simulink library "Brakes_Axle2_HydraulicValves_Channel4"  (R2026a)
settings: Solver=VariableStepAuto
undefined symbols (not defined in the file): Brakes
libraries: fl_lib x32, nesl_utility x18, SimscapeFluids_lib x8, sdl_lib x4, Brakes_Elements x4
(part 1 of 2)
Description:
  | Component of Simscape Vehicle Templates Library
  | 
  | Copyright 2018-2026 The MathWorks, Inc.
settings Model: Creator=smiller  LastModifiedBy=smiller

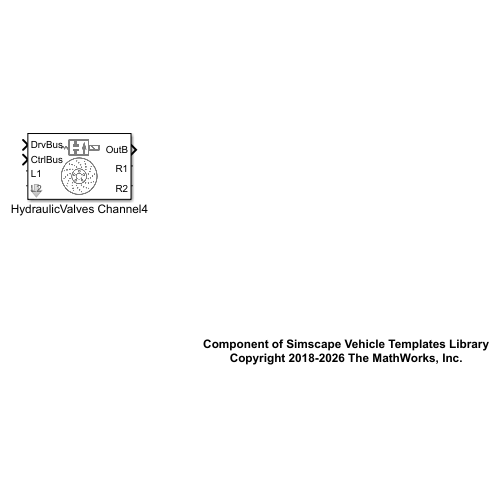
[thumbnail: Simulink's stored preview of the top-level diagram]
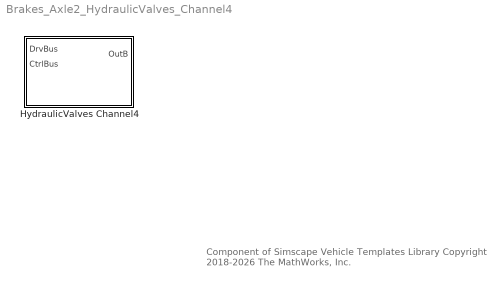
== system Brakes_Axle2_HydraulicValves_Channel4 ==
  note: Component of Simscape Vehicle Templates Library
      | Copyright 2018-2026 The MathWorks, Inc.
  HydraulicValves Channel4 : Subsystem  Tag=PublishSubsystem  VariantControl=ABS_4_Channel  mask(Four Channel ABS){d_caliper_bore_a1=Brakes.Axle1.Caliper.lCylinderDiameter.Value, d_caliper_bore_a2=Brakes.Axle2.Caliper.lCylinderDiameter.Value, brk_pad_rad_a1=Brakes.Axle1.DiscAndPad.lMeanRadius.Value, brk_pad_rad_a2=Brakes.Axle2.DiscAndPad.lMeanRadius.Value, brk_cyl_bore_a1=Brakes.Axle1.Caliper.lCylinderDiameter.Value, brk_cyl_bore_a2=Brakes.Axle2.Caliper.lCylinderDiameter.Value, brk_n_pads_a1=Brakes.Axle1.DiscAndPad.NPads.Value, brk_n_pads_a2=Brakes.Axle2.DiscAndPad.NPads.Value, brk_mu_static_a1=Brakes.Axle1.DiscAndPad.rMuStatic.Value, brk_mu_static_a2=Brakes.Axle2.DiscAndPad.rMuStatic.Value, brk_mu_kin_a1=Brakes.Axle1.DiscAndPad.rMuKinetic.Value, brk_mu_kin_a2=Brakes.Axle2.DiscAndPad.rMuKinetic.Value, brk_trans_vel_a1=Brakes.Axle1.DiscAndPad.nTransition.Value, brk_trans_vel_a2=Brakes.Axle2.DiscAndPad.nTransition.Value, brk_visc_coef_a1=Brakes.Axle1.DiscAndPad.dViscous.Value, brk_visc_coef_a2=Brakes.Axle2.DiscAndPad.dViscous.Value, spr_rate=Brakes.Axle1.ValveApply.kSpring.Value, D=Brakes.Axle1.ValveApply.bDamper.Value, area_max_apply=Brakes.Axle1.ValveApply.AMax.Value, open_max_apply=Brakes.Axle1.ValveApply.xMax.Value, area_max_rel=Brakes.Axle1.ValveRelease.AMax.Value, open_max_rel=Brakes.Axle1.ValveRelease.xMax.Value, p_max_a1=Brakes.Axle1.Caliper.pMax.Value, p_max_a2=Brakes.Axle2.Caliper.pMax.Value, brkTs=Brakes.Axle1.ValveApply.fValveTime.Value}
      mask prompts: spr_rate "Spring Rate (N/m)"; D "Damping coefficient"; area_max_apply "Max Area Apply Valve (m^2)"; open_max_apply "Max Opening Apply Valve (m)"; area_max_rel "Max Area Release Valve (m^2)"; open_max_rel "Max Opening Release Valve (m)"; p_max_a1 "Max Master Cylinder Pressure Axle 1 (bar)"; p_max_a2 "Max Master Cylinder Pressure Axle 2 (bar)"; brkTs "Filter time constant"
      mask help: Models braking system for four wheels. Valve signals control hydraulic pressure at each wheel individually.
      mask init:
      | pist_area_pist_a1 = pi*d_caliper_bore_a1^2/4;
      | pist_area_pist_a2 = pi*d_caliper_bore_a2^2/4;
      mask TypeOptions brk_pad_rad_a1:
      | Disc
      | Brake
      | L1/r_mean | Disc
      | Brake
      | R1/r_mean
      mask TypeOptions brk_pad_rad_a2:
      | Disc
      | Brake
      | L2/r_mean | Disc
      | Brake
      | R2/r_mean
      mask TypeOptions brk_cyl_bore_a1:
      | Disc
      | Brake
      | L1/bore | Disc
      | Brake
      | R1/bore
      mask TypeOptions brk_cyl_bore_a2:
      | Disc
      | Brake
      | L2/bore | Disc
      | Brake
      | R2/bore
      mask TypeOptions brk_n_pads_a1:
      | Disc
      | Brake
      | L1/n_pads | Disc
      | Brake
      | R1/n_pads
      mask TypeOptions brk_n_pads_a2:
      | Disc
      | Brake
      | L2/n_pads | Disc
      | Brake
      | R2/n_pads
      mask TypeOptions brk_mu_static_a1:
      | Disc
      | Brake
      | L1/mu_static | Disc
      | Brake
      | R1/mu_static
      mask TypeOptions brk_mu_static_a2:
      | Disc
      | Brake
      | L2/mu_static | Disc
      | Brake
      | R2/mu_static
      mask TypeOptions brk_mu_kin_a1:
      | Disc
      | Brake
      | L1/mu_coulomb | Disc
      | Brake
      | R1/mu_coulomb
      mask TypeOptions brk_mu_kin_a2:
      | Disc
      | Brake
      | L2/mu_coulomb | Disc
      | Brake
      | R2/mu_coulomb
      mask TypeOptions brk_trans_vel_a1:
      | Disc
      | Brake
      | L1/brkwy_vel | Disc
      | Brake
      | R1/brkwy_vel
      mask TypeOptions brk_trans_vel_a2:
      | Disc
      | Brake
      | L2/brkwy_vel | Disc
      | Brake
      | R2/brkwy_vel
      mask TypeOptions brk_visc_coef_a1:
      | Disc
      | Brake
      | L1/visc_coef
      mask TypeOptions brk_visc_coef_a2:
      | Disc
      | Brake
      | L2/visc_coef | Disc
      | Brake
      | R2/visc_coef
      mask TypeOptions spr_rate: Valves/spr_rate
      mask TypeOptions D: Valves/D
      mask TypeOptions area_max_apply: Valves/area_max_apply
      mask TypeOptions open_max_apply: Valves/open_max_apply
      mask TypeOptions area_max_rel: Valves/area_max_rel
      mask TypeOptions open_max_rel: Valves/open_max_rel
      mask TypeOptions p_max_a1: Valves/p_max_a1
      mask TypeOptions p_max_a2: Valves/p_max_a2
      mask TypeOptions brkTs: Valves/brkTs
      mask DialogControl Container10 Prompt: Geometry
      mask DialogControl cont_brk_geom Prompt: Geometry
      mask DialogControl text_brakes_a1 Prompt: Axle 1
      mask DialogControl text_brakes_a2 Prompt: Axle 2
      mask DialogControl text_caliper_bore Prompt: Caliper Bore (m)
      mask DialogControl text_brakes_pad_rad Prompt: Mean Pad Radius (m)
      mask DialogControl text_brakes_cyl_bore Prompt: Cylinder Bore (m)
      mask DialogControl text_brakes_n_pads Prompt: Number of pads
      mask DialogControl Container9 Prompt: Friction
      mask DialogControl cont_brk_frict Prompt: Friction
      mask DialogControl text_brakes_mu_static Prompt: Static Coeff. (0-1)
      mask DialogControl text_brakes_mu_kin Prompt: Kinetic Coeff. (0-1)
      mask DialogControl text_brakes_trans_vel Prompt: Trans. Velocity (rad/s)
      mask DialogControl text_brakes_visc_coef Prompt: Viscous (N*m/(rad/s))
      mask DialogControl cont_valves Prompt: Valves
      mask Display: image('sm_car_vehicle_brakes_abs_IMAGE.png');

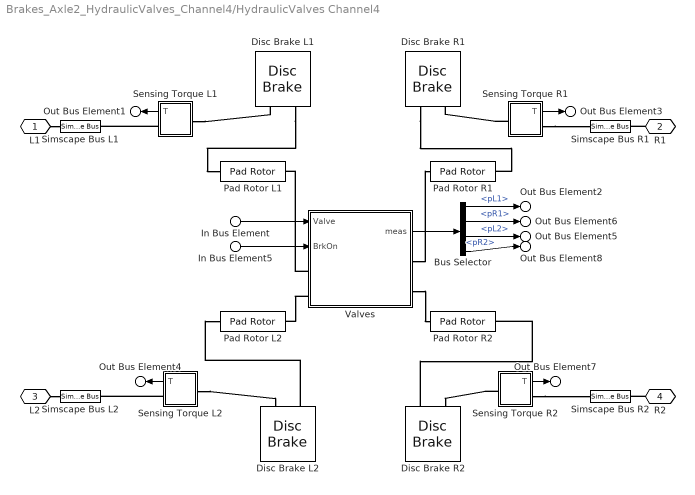
== system Brakes_Axle2_HydraulicValves_Channel4/HydraulicValves Channel4 ==
  In Bus Element5 : Inport  PortName=DrvBus  Element=rBrakePedal
  In Bus Element : Inport  Port=2  PortName=CtrlBus  Element=Valves
  Bus Selector : BusSelector  OutputSignals=pL1,pR1,pL2,pR2
  Disc Brake L1 : sdl_lib/Brakes & Detents/Rotational/Disc Brake  r_mean=brk_pad_rad_a1 m  bore=brk_cyl_bore_a1 m  n_pads=brk_n_pads_a1  thermal_port=simscape.enum.thermaleffects.omit  mu_static=brk_mu_static_a1  mu_coulomb=brk_mu_kin_a1  temperature_TLU=[280, 300, 320] K  mu_static_TLU=[.9, .8, .7]  mu_coulomb_TLU=[.8, .7, .6]  brkwy_vel=brk_trans_vel_a1 rad/s  visc_coef=brk_visc_coef_a1 N*m/(rad/s)  thermal_mass=50 kJ/K  temperature_specify=off  temperature_priority=High  temperature=300 K  temperature_nominal_specify=off  temperature_nominal_value=1  temperature_nominal_unit=K
  Disc Brake L2 : sdl_lib/Brakes & Detents/Rotational/Disc Brake  r_mean=brk_pad_rad_a2 m  bore=brk_cyl_bore_a2 m  n_pads=brk_n_pads_a2  thermal_port=simscape.enum.thermaleffects.omit  mu_static=brk_mu_static_a2  mu_coulomb=brk_mu_kin_a2  temperature_TLU=[280, 300, 320] K  mu_static_TLU=[.9, .8, .7]  mu_coulomb_TLU=[.8, .7, .6]  brkwy_vel=brk_trans_vel_a2 rad/s  visc_coef=brk_visc_coef_a2 N*m/(rad/s)  thermal_mass=50 kJ/K  temperature_specify=off  temperature_priority=High  temperature=300 K  temperature_nominal_specify=off  temperature_nominal_value=1  temperature_nominal_unit=K
  Disc Brake R1 : sdl_lib/Brakes & Detents/Rotational/Disc Brake  r_mean=brk_pad_rad_a1 m  bore=brk_cyl_bore_a1 m  n_pads=brk_n_pads_a1  thermal_port=simscape.enum.thermaleffects.omit  mu_static=brk_mu_static_a1  mu_coulomb=brk_mu_kin_a1  temperature_TLU=[280, 300, 320] K  mu_static_TLU=[.9, .8, .7]  mu_coulomb_TLU=[.8, .7, .6]  brkwy_vel=brk_trans_vel_a1 rad/s  visc_coef=.001 N*m/(rad/s)  thermal_mass=50 kJ/K  temperature_specify=off  temperature_priority=High  temperature=300 K  temperature_nominal_specify=off  temperature_nominal_value=1  temperature_nominal_unit=K
  Disc Brake R2 : sdl_lib/Brakes & Detents/Rotational/Disc Brake  r_mean=brk_pad_rad_a2 m  bore=brk_cyl_bore_a2 m  n_pads=brk_n_pads_a2  thermal_port=simscape.enum.thermaleffects.omit  mu_static=brk_mu_static_a2  mu_coulomb=brk_mu_kin_a2  temperature_TLU=[280, 300, 320] K  mu_static_TLU=[.9, .8, .7]  mu_coulomb_TLU=[.8, .7, .6]  brkwy_vel=brk_trans_vel_a2 rad/s  visc_coef=brk_visc_coef_a2 N*m/(rad/s)  thermal_mass=50 kJ/K  temperature_specify=off  temperature_priority=High  temperature=300 K  temperature_nominal_specify=off  temperature_nominal_value=1  temperature_nominal_unit=K
  Pad Rotor L1 : Brakes_Elements/Pad Rotor  d_caliper_piston_f=d_caliper_bore_a1
  Pad Rotor L2 : Brakes_Elements/Pad Rotor  d_caliper_piston_f=d_caliper_bore_a2
  Pad Rotor R1 : Brakes_Elements/Pad Rotor  d_caliper_piston_f=d_caliper_bore_a1
  Pad Rotor R2 : Brakes_Elements/Pad Rotor  d_caliper_piston_f=d_caliper_bore_a2
  Sensing Torque L1 : Subsystem
  Sensing Torque L2 : Subsystem
  Sensing Torque R1 : Subsystem
  Sensing Torque R2 : Subsystem
  Simscape Bus L1 : SimscapeBus  HierarchyStrings=Axle1D
  Simscape Bus L2 : SimscapeBus  HierarchyStrings=Axle1D
  Simscape Bus R1 : SimscapeBus  HierarchyStrings=Axle1D
  Simscape Bus R2 : SimscapeBus  HierarchyStrings=Axle1D
  Valves : Subsystem  VariantControl=Valves  mask{brkTs=brkTs, p_max_a1=p_max_a1, p_max_a2=p_max_a2, spr_rate=spr_rate, D=D, area_max_apply=area_max_apply, open_max_apply=open_max_apply, area_max_rel=area_max_rel, open_max_rel=open_max_rel}
      mask prompts: brkTs "Filter time constant"; p_max_a1 "Max Pressure Axle 1 (bar)"; p_max_a2 "Max Pressure Axle 2 (bar)"; spr_rate "Spring Rate (N/m)"; D "Damping coefficient"; area_max_apply "Max Area Apply Valve (m^2)"; open_max_apply "Max Opening Apply Valve (m)"; area_max_rel "Max Area Release Valve (m^2)"; open_max_rel "Max Opening Release Valve (m)"
      mask TypeOptions brkTs:
      | Valves L1/Actuator
      | Dynamics/b | Valves R1/Actuator
      | Dynamics/b | Valves L2/Actuator
      | Dynamics/b | Valves R2/Actuator
      | Dynamics/b
      mask TypeOptions p_max_a1: MC Pressure A1/Value
      mask TypeOptions p_max_a2: MC Pressure A2/Value
      mask TypeOptions spr_rate: Return Spring L1/Spring/spr_rate | Return Spring R1/Spring/spr_rate | Return Spring L2/Spring/spr_rate | Return Spring R2/Spring/spr_rate
      mask TypeOptions D: Return Spring L1/Damper/D | Return Spring R1/Damper/D | Return Spring L2/Damper/D | Return Spring R2/Damper/D
  L1 : PMIOPort  Side=Left
  R1 : PMIOPort  Port=2  Side=Right
  L2 : PMIOPort  Port=3  Side=Left
  R2 : PMIOPort  Port=4  Side=Right
  Out Bus Element1 : Outport  VectorParamsAs1DForOutWhenUnconnected=off  PortName=OutB  Element=MBrakeL1
  Out Bus Element3 : Outport  VectorParamsAs1DForOutWhenUnconnected=off  PortName=OutB  Element=MBrakeR1
  Out Bus Element4 : Outport  VectorParamsAs1DForOutWhenUnconnected=off  PortName=OutB  Element=MBrakeL2
  Out Bus Element7 : Outport  VectorParamsAs1DForOutWhenUnconnected=off  PortName=OutB  Element=MBrakeR2
  Out Bus Element2 : Outport  VectorParamsAs1DForOutWhenUnconnected=off  PortName=OutB  Element=pBrakeL1
  Out Bus Element6 : Outport  VectorParamsAs1DForOutWhenUnconnected=off  PortName=OutB  Element=pBrakeR1
  Out Bus Element5 : Outport  VectorParamsAs1DForOutWhenUnconnected=off  PortName=OutB  Element=pBrakeL2
  Out Bus Element8 : Outport  VectorParamsAs1DForOutWhenUnconnected=off  PortName=OutB  Element=pBrakeR2
  wires:
  Sensing Torque L1/1(T) -> Out Bus Element1/1
  Bus Selector/4 -> Out Bus Element8/1  "<pR2>"
  Sensing Torque R1/1(T) -> Out Bus Element3/1
  Sensing Torque R2/1(T) -> Out Bus Element7/1
  Bus Selector/2 -> Out Bus Element6/1  "<pR1>"
  Bus Selector/1 -> Out Bus Element2/1  "<pL1>"
  Sensing Torque L2/1(T) -> Out Bus Element4/1
  Bus Selector/3 -> Out Bus Element5/1  "<pL2>"
  Valves/1(meas) -> Bus Selector/1
  In Bus Element/1 -> Valves/1(Valve)
  In Bus Element5/1 -> Valves/2(BrkOn)
  connections:
  Sensing Torque L2/RConn1 -- Simscape Bus L2/LConn1
  Valves/LConn2 -- Pad Rotor L2/RConn1
  Disc Brake R1/LConn1 -- Pad Rotor R1/LConn1
  Sensing Torque R1/LConn1 -- Disc Brake R1/LConn2
  Disc Brake R2/LConn1 -- Pad Rotor R2/LConn1
  Valves/RConn2 -- Pad Rotor R2/RConn1
  L2/RConn1 -- Simscape Bus L2/RConn1
  Sensing Torque R2/LConn1 -- Disc Brake R2/LConn2
  Sensing Torque R1/RConn1 -- Simscape Bus R1/LConn1
  Disc Brake L2/LConn1 -- Pad Rotor L2/LConn1
  Sensing Torque R2/RConn1 -- Simscape Bus R2/LConn1
  Sensing Torque L1/RConn1 -- Simscape Bus L1/LConn1
  Sensing Torque L1/LConn1 -- Disc Brake L1/LConn2
  R2/RConn1 -- Simscape Bus R2/RConn1
  R1/RConn1 -- Simscape Bus R1/RConn1
  Sensing Torque L2/LConn1 -- Disc Brake L2/LConn2
  Valves/LConn1 -- Pad Rotor L1/RConn1
  Disc Brake L1/LConn1 -- Pad Rotor L1/LConn1
  L1/RConn1 -- Simscape Bus L1/RConn1
  Valves/RConn1 -- Pad Rotor R1/RConn1

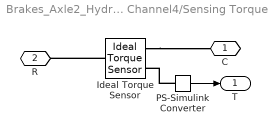
== system Brakes_Axle2_HydraulicValves_Channel4/HydraulicValves Channel4/Sensing Torque L1 ==
  Ideal Torque Sensor : fl_lib/Mechanical/Mechanical Sensors/Ideal Torque Sensor
  PS-Simulink Converter : nesl_utility/PS-Simulink Converter  PhysicalDomain=network_engine_domain  SubClassName=ps_output  LeftPortType=input  RightPortType=output  PseudoPeriodic=off  Frequencies=[]  VectorFormat=1-D array  Unit=N*m  AffineConversion=off
  C : PMIOPort  Side=Right
  R : PMIOPort  Port=2  Side=Left
  T : Outport  VectorParamsAs1DForOutWhenUnconnected=off
  wires:
  PS-Simulink Converter/1 -> T/1
  connections:
  Ideal Torque Sensor/LConn1 -- R/RConn1
  Ideal Torque Sensor/RConn1 -- C/RConn1
  PS-Simulink Converter/LConn1 -- Ideal Torque Sensor/RConn2

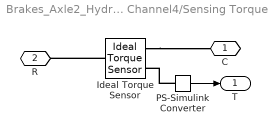
== system Brakes_Axle2_HydraulicValves_Channel4/HydraulicValves Channel4/Sensing Torque L2 ==
  Ideal Torque Sensor : fl_lib/Mechanical/Mechanical Sensors/Ideal Torque Sensor
  PS-Simulink Converter : nesl_utility/PS-Simulink Converter  PhysicalDomain=network_engine_domain  SubClassName=ps_output  LeftPortType=input  RightPortType=output  PseudoPeriodic=off  Frequencies=[]  VectorFormat=1-D array  Unit=N*m  AffineConversion=off
  C : PMIOPort  Side=Right
  R : PMIOPort  Port=2  Side=Left
  T : Outport  VectorParamsAs1DForOutWhenUnconnected=off
  wires:
  PS-Simulink Converter/1 -> T/1
  connections:
  PS-Simulink Converter/LConn1 -- Ideal Torque Sensor/RConn2
  Ideal Torque Sensor/RConn1 -- C/RConn1
  Ideal Torque Sensor/LConn1 -- R/RConn1

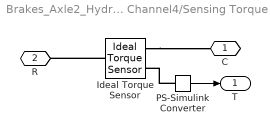
== system Brakes_Axle2_HydraulicValves_Channel4/HydraulicValves Channel4/Sensing Torque R1 ==
  Ideal Torque Sensor : fl_lib/Mechanical/Mechanical Sensors/Ideal Torque Sensor
  PS-Simulink Converter : nesl_utility/PS-Simulink Converter  PhysicalDomain=network_engine_domain  SubClassName=ps_output  LeftPortType=input  RightPortType=output  PseudoPeriodic=off  Frequencies=[]  VectorFormat=1-D array  Unit=N*m  AffineConversion=off
  C : PMIOPort  Side=Right
  R : PMIOPort  Port=2  Side=Left
  T : Outport  VectorParamsAs1DForOutWhenUnconnected=off
  wires:
  PS-Simulink Converter/1 -> T/1
  connections:
  Ideal Torque Sensor/LConn1 -- R/RConn1
  Ideal Torque Sensor/RConn1 -- C/RConn1
  PS-Simulink Converter/LConn1 -- Ideal Torque Sensor/RConn2

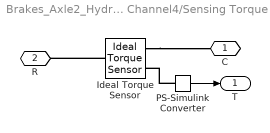
== system Brakes_Axle2_HydraulicValves_Channel4/HydraulicValves Channel4/Sensing Torque R2 ==
  Ideal Torque Sensor : fl_lib/Mechanical/Mechanical Sensors/Ideal Torque Sensor
  PS-Simulink Converter : nesl_utility/PS-Simulink Converter  PhysicalDomain=network_engine_domain  SubClassName=ps_output  LeftPortType=input  RightPortType=output  PseudoPeriodic=off  Frequencies=[]  VectorFormat=1-D array  Unit=N*m  AffineConversion=off
  C : PMIOPort  Side=Right
  R : PMIOPort  Port=2  Side=Left
  T : Outport  VectorParamsAs1DForOutWhenUnconnected=off
  wires:
  PS-Simulink Converter/1 -> T/1
  connections:
  PS-Simulink Converter/LConn1 -- Ideal Torque Sensor/RConn2
  Ideal Torque Sensor/RConn1 -- C/RConn1
  Ideal Torque Sensor/LConn1 -- R/RConn1

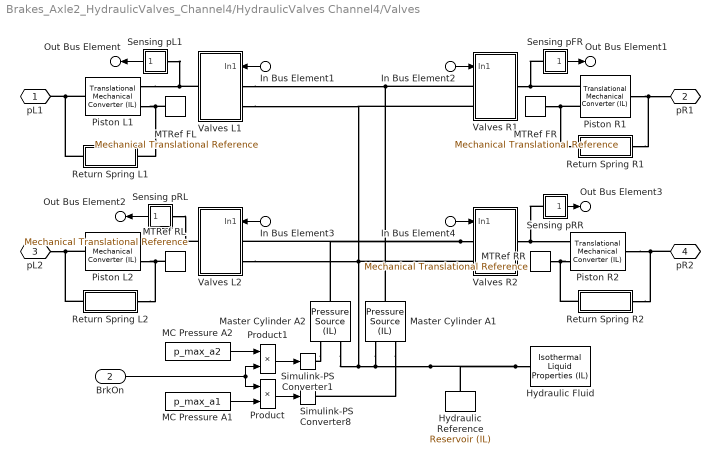
== system Brakes_Axle2_HydraulicValves_Channel4/HydraulicValves Channel4/Valves ==
  In Bus Element1 : Inport  PortName=Valve  Element=L1
  In Bus Element2 : Inport  PortName=Valve  Element=R1
  In Bus Element3 : Inport  PortName=Valve  Element=L2
  In Bus Element4 : Inport  PortName=Valve  Element=R2
  BrkOn : Inport  Port=2
  Hydraulic Fluid : fl_lib/Isothermal Liquid/Utilities/Isothermal Liquid Properties (IL)  rho_L_atm=1001.952 kg/m^3  bulk_modulus_model=foundation.enum.bulk_modulus_model.const  beta_gain=6  beta_L_atm=1.52340e+09 Pa  nu_atm=(2.786)*(1) cSt  p_atm=0.101325 MPa  p_min=0.1 Pa  properties_range_check=simscape.enum.assert.action.error  air_fraction=0.005  polytropic_index=1.0  rho_g_atm=1.225 kg/m^3  air_dissolution_model=simscape.enum.onoff.off  p_crit=3 MPa
      settings: LibrarySourceBlock=sh_lib/Hydraulic Utilities/Hydraulic Fluid
  Hydraulic Reference : fl_lib/Isothermal Liquid/Elements/Reservoir (IL)  pressure_input=false  pressure_spec=foundation.enum.pressure_spec.atmospheric  reservoir_pressure=0.101325 MPa
      settings: LibrarySourceBlock=fl_lib/Hydraulic/Hydraulic Elements/Hydraulic Reference
  MC Pressure A1 : Constant  Value=p_max_a1
  MC Pressure A2 : Constant  Value=p_max_a2
  MTRef FL : fl_lib/Mechanical/Translational Elements/Mechanical Translational Reference
  MTRef FR : fl_lib/Mechanical/Translational Elements/Mechanical Translational Reference
  MTRef RL : fl_lib/Mechanical/Translational Elements/Mechanical Translational Reference
  MTRef RR : fl_lib/Mechanical/Translational Elements/Mechanical Translational Reference
  Master Cylinder A1 : fl_lib/Isothermal Liquid/Sources/Pressure Source (IL)  source_type=foundation.enum.constant_controlled.controlled  pressure_differential=0 MPa
      settings: LibrarySourceBlock=|
      | fl_lib/Hydraulic/Hydraulic Sources/Hydraulic Pressure
      | Source
  Master Cylinder A2 : fl_lib/Isothermal Liquid/Sources/Pressure Source (IL)  source_type=foundation.enum.constant_controlled.controlled  pressure_differential=0 MPa
      settings: LibrarySourceBlock=|
      | fl_lib/Hydraulic/Hydraulic Sources/Hydraulic Pressure
      | Source
  Piston L1 : fl_lib/Isothermal Liquid/Elements/Translational Mechanical Converter (IL)  mech_orientation=1  displacement_spec=foundation.enum.DisplacementSpec.Calculate  x0=0 m  interface_area=pist_area_pist_a1 m^2  dead_volume=1e-4 m^3  pressure_spec=1  environment_pressure=0.101325 MPa  dynamic_compressibility=1  p0=0 + 101325 Pa  p_nominal=0.101325 MPa
      settings: LibrarySourceBlock=|
      | fl_lib/Hydraulic/Hydraulic Elements/Translational
      | Hydro-Mechanical
      | Converter
  Piston L2 : fl_lib/Isothermal Liquid/Elements/Translational Mechanical Converter (IL)  mech_orientation=1  displacement_spec=foundation.enum.DisplacementSpec.Calculate  x0=0 m  interface_area=pist_area_pist_a2 m^2  dead_volume=1e-4 m^3  pressure_spec=1  environment_pressure=0.101325 MPa  dynamic_compressibility=1  p0=0 + 101325 Pa  p_nominal=0.101325 MPa
      settings: LibrarySourceBlock=|
      | fl_lib/Hydraulic/Hydraulic Elements/Translational
      | Hydro-Mechanical
      | Converter
  Piston R1 : fl_lib/Isothermal Liquid/Elements/Translational Mechanical Converter (IL)  mech_orientation=1  displacement_spec=foundation.enum.DisplacementSpec.Calculate  x0=0 m  interface_area=pist_area_pist_a1 m^2  dead_volume=1e-4 m^3  pressure_spec=1  environment_pressure=0.101325 MPa  dynamic_compressibility=1  p0=0 + 101325 Pa  p_nominal=0.101325 MPa
      settings: LibrarySourceBlock=|
      | fl_lib/Hydraulic/Hydraulic Elements/Translational
      | Hydro-Mechanical
      | Converter
  Piston R2 : fl_lib/Isothermal Liquid/Elements/Translational Mechanical Converter (IL)  mech_orientation=1  displacement_spec=foundation.enum.DisplacementSpec.Calculate  x0=0 m  interface_area=pist_area_pist_a2 m^2  dead_volume=1e-4 m^3  pressure_spec=1  environment_pressure=0.101325 MPa  dynamic_compressibility=1  p0=0 + 101325 Pa  p_nominal=0.101325 MPa
      settings: LibrarySourceBlock=|
      | fl_lib/Hydraulic/Hydraulic Elements/Translational
      | Hydro-Mechanical
      | Converter
  Product : Product
  Product1 : Product
  Return Spring L1 : Subsystem
  Return Spring L2 : Subsystem
  Return Spring R1 : Subsystem
  Return Spring R2 : Subsystem
  Sensing pFR : Subsystem
  Sensing pL1 : Subsystem
  Sensing pRL : Subsystem
  Sensing pRR : Subsystem
  Simulink-PS Converter1 : nesl_utility/Simulink-PS Converter  PhysicalDomain=network_engine_domain  SubClassName=ps_input  LeftPortType=input  RightPortType=output  PseudoPeriodic=off  Frequencies=[]  NoiseDistribution=none  NoiseParameters=[]  Unit=bar  AffineConversion=off  FilteringAndDerivatives=provide  SimscapeFilterOrder=1  InputFilterTimeConstant=0.001  UdotUserProvided=0
  Simulink-PS Converter8 : nesl_utility/Simulink-PS Converter  PhysicalDomain=network_engine_domain  SubClassName=ps_input  LeftPortType=input  RightPortType=output  PseudoPeriodic=off  Frequencies=[]  NoiseDistribution=none  NoiseParameters=[]  Unit=bar  AffineConversion=off  FilteringAndDerivatives=provide  SimscapeFilterOrder=1  InputFilterTimeConstant=0.001  UdotUserProvided=0
  Valves L1 : Subsystem
  Valves L2 : Subsystem
  Valves R1 : Subsystem
  Valves R2 : Subsystem
  pL1 : PMIOPort  Side=Left
  pR1 : PMIOPort  Port=2  Side=Right
  pL2 : PMIOPort  Port=3  Side=Left
  pR2 : PMIOPort  Port=4  Side=Right
  Out Bus Element : Outport  VectorParamsAs1DForOutWhenUnconnected=off  PortName=meas  Element=pL1
  Out Bus Element1 : Outport  VectorParamsAs1DForOutWhenUnconnected=off  PortName=meas  Element=pR1
  Out Bus Element2 : Outport  VectorParamsAs1DForOutWhenUnconnected=off  PortName=meas  Element=pL2
  Out Bus Element3 : Outport  VectorParamsAs1DForOutWhenUnconnected=off  PortName=meas  Element=pR2
  wires:
  Product/1 -> Simulink-PS Converter8/1
  BrkOn/1 -> Product/1, Product1/2
  In Bus Element3/1 -> Valves L2/1(In1)
  In Bus Element4/1 -> Valves R2/1(In1)
  In Bus Element2/1 -> Valves R1/1(In1)
  In Bus Element1/1 -> Valves L1/1(In1)
  MC Pressure A1/1 -> Product/2
  Sensing pRL/1(p) -> Out Bus Element2/1
  Sensing pRR/1(p) -> Out Bus Element3/1
  Sensing pFR/1(p) -> Out Bus Element1/1
  Sensing pL1/1(p) -> Out Bus Element/1
  Product1/1 -> Simulink-PS Converter1/1
  MC Pressure A2/1 -> Product1/1
  connections:
  MTRef FR/LConn1 -- Return Spring R1/LConn1 -- Piston R1/LConn2
  MTRef FL/LConn1 -- Return Spring L1/LConn1 -- Piston L1/LConn2
  MTRef RL/LConn1 -- Return Spring L2/LConn1 -- Piston L2/LConn2
  Valves R1/LConn1 -- Master Cylinder A1/RConn1 -- Valves L1/LConn1
  Hydraulic Fluid/RConn1 -- Master Cylinder A1/LConn1 -- Master Cylinder A2/LConn1 -- Valves R2/LConn2 -- Valves R1/LConn2 -- Valves L1/LConn2 -- Valves L2/LConn2 -- Hydraulic Reference/LConn1
  Return Spring R1/RConn1 -- Piston R1/RConn1 -- pR1/RConn1
  Sensing pRR/LConn1 -- Valves R2/RConn1 -- Piston R2/LConn1
  Sensing pFR/LConn1 -- Valves R1/RConn1 -- Piston R1/LConn1
  Master Cylinder A1/LConn2 -- Simulink-PS Converter8/RConn1
  Valves R2/LConn1 -- Master Cylinder A2/RConn1 -- Valves L2/LConn1
  Master Cylinder A2/LConn2 -- Simulink-PS Converter1/RConn1
  Valves L1/RConn1 -- Sensing pL1/LConn1 -- Piston L1/LConn1
  Return Spring L1/RConn1 -- Piston L1/RConn1 -- pL1/RConn1
  Return Spring L2/RConn1 -- pL2/RConn1 -- Piston L2/RConn1
  Sensing pRL/LConn1 -- Piston L2/LConn1 -- Valves L2/RConn1
  Return Spring R2/LConn1 -- MTRef RR/LConn1 -- Piston R2/LConn2
  pR2/RConn1 -- Piston R2/RConn1 -- Return Spring R2/RConn1

== system Brakes_Axle2_HydraulicValves_Channel4/HydraulicValves Channel4/Valves/Return Spring L1 ==
  Damper : fl_lib/Mechanical/Translational Elements/Translational Damper  D=D N/(m/s)  v_specify=off  v_priority=None  v=0 m/s  v_nominal_specify=off  v_nominal_value=1  v_nominal_unit=m/s  f_specify=off  f_priority=None  f=0 N  f_nominal_specify=off  f_nominal_value=1  f_nominal_unit=N
  Spring : fl_lib/Mechanical/Translational Elements/Translational Spring  spr_rate=spr_rate N/m  v_specify=off  v_priority=None  v=0 m/s  v_nominal_specify=off  v_nominal_value=1  v_nominal_unit=m/s  f_specify=off  f_priority=None  f=0 N  f_nominal_specify=off  f_nominal_value=1  f_nominal_unit=N  x_specify=off  x_priority=High  x=0 m  x_nominal_specify=off  x_nominal_value=1  x_nominal_unit=m
  R : PMIOPort  Side=Right
  C : PMIOPort  Port=2  Side=Left
  connections:
  Spring/RConn1 -- Damper/RConn1 -- C/RConn1
  Spring/LConn1 -- R/RConn1 -- Damper/LConn1

== system Brakes_Axle2_HydraulicValves_Channel4/HydraulicValves Channel4/Valves/Return Spring L2 ==
  Damper : fl_lib/Mechanical/Translational Elements/Translational Damper  D=D N/(m/s)  v_specify=off  v_priority=None  v=0 m/s  v_nominal_specify=off  v_nominal_value=1  v_nominal_unit=m/s  f_specify=off  f_priority=None  f=0 N  f_nominal_specify=off  f_nominal_value=1  f_nominal_unit=N
  Spring : fl_lib/Mechanical/Translational Elements/Translational Spring  spr_rate=spr_rate N/m  v_specify=off  v_priority=None  v=0 m/s  v_nominal_specify=off  v_nominal_value=1  v_nominal_unit=m/s  f_specify=off  f_priority=None  f=0 N  f_nominal_specify=off  f_nominal_value=1  f_nominal_unit=N  x_specify=off  x_priority=High  x=0 m  x_nominal_specify=off  x_nominal_value=1  x_nominal_unit=m
  R : PMIOPort  Side=Right
  C : PMIOPort  Port=2  Side=Left
  connections:
  R/RConn1 -- Damper/LConn1 -- Spring/LConn1
  C/RConn1 -- Spring/RConn1 -- Damper/RConn1

== system Brakes_Axle2_HydraulicValves_Channel4/HydraulicValves Channel4/Valves/Return Spring R1 ==
  Damper : fl_lib/Mechanical/Translational Elements/Translational Damper  D=D N/(m/s)  v_specify=off  v_priority=None  v=0 m/s  v_nominal_specify=off  v_nominal_value=1  v_nominal_unit=m/s  f_specify=off  f_priority=None  f=0 N  f_nominal_specify=off  f_nominal_value=1  f_nominal_unit=N
  Spring : fl_lib/Mechanical/Translational Elements/Translational Spring  spr_rate=spr_rate N/m  v_specify=off  v_priority=None  v=0 m/s  v_nominal_specify=off  v_nominal_value=1  v_nominal_unit=m/s  f_specify=off  f_priority=None  f=0 N  f_nominal_specify=off  f_nominal_value=1  f_nominal_unit=N  x_specify=off  x_priority=High  x=0 m  x_nominal_specify=off  x_nominal_value=1  x_nominal_unit=m
  R : PMIOPort  Side=Right
  C : PMIOPort  Port=2  Side=Left
  connections:
  Damper/LConn1 -- R/RConn1 -- Spring/LConn1
  C/RConn1 -- Damper/RConn1 -- Spring/RConn1

== system Brakes_Axle2_HydraulicValves_Channel4/HydraulicValves Channel4/Valves/Return Spring R2 ==
  Damper : fl_lib/Mechanical/Translational Elements/Translational Damper  D=D N/(m/s)  v_specify=off  v_priority=None  v=0 m/s  v_nominal_specify=off  v_nominal_value=1  v_nominal_unit=m/s  f_specify=off  f_priority=None  f=0 N  f_nominal_specify=off  f_nominal_value=1  f_nominal_unit=N
  Spring : fl_lib/Mechanical/Translational Elements/Translational Spring  spr_rate=spr_rate N/m  v_specify=off  v_priority=None  v=0 m/s  v_nominal_specify=off  v_nominal_value=1  v_nominal_unit=m/s  f_specify=off  f_priority=None  f=0 N  f_nominal_specify=off  f_nominal_value=1  f_nominal_unit=N  x_specify=off  x_priority=High  x=0 m  x_nominal_specify=off  x_nominal_value=1  x_nominal_unit=m
  R : PMIOPort  Side=Right
  C : PMIOPort  Port=2  Side=Left
  connections:
  Spring/RConn1 -- Damper/RConn1 -- C/RConn1
  Spring/LConn1 -- R/RConn1 -- Damper/LConn1

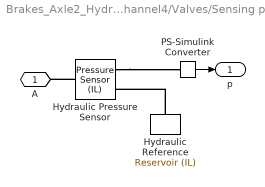
== system Brakes_Axle2_HydraulicValves_Channel4/HydraulicValves Channel4/Valves/Sensing pFR ==
  Hydraulic Pressure Sensor : fl_lib/Isothermal Liquid/Sensors/Pressure Sensor (IL)  pressure_measure=foundation.enum.pressure_measure.difference
      settings: LibrarySourceBlock=|
      | fl_lib/Hydraulic/Hydraulic Sensors/Hydraulic Pressure
      | Sensor
  Hydraulic Reference : fl_lib/Isothermal Liquid/Elements/Reservoir (IL)  pressure_input=false  pressure_spec=foundation.enum.pressure_spec.atmospheric  reservoir_pressure=0.101325 MPa
      settings: LibrarySourceBlock=fl_lib/Hydraulic/Hydraulic Elements/Hydraulic Reference
  PS-Simulink Converter : nesl_utility/PS-Simulink Converter  PhysicalDomain=network_engine_domain  SubClassName=ps_output  LeftPortType=input  RightPortType=output  PseudoPeriodic=off  Frequencies=[]  VectorFormat=1-D array  Unit=bar  AffineConversion=off
  A : PMIOPort  Side=Left
  p : Outport  VectorParamsAs1DForOutWhenUnconnected=off
  wires:
  PS-Simulink Converter/1 -> p/1
  connections:
  Hydraulic Pressure Sensor/RConn2 -- PS-Simulink Converter/LConn1
  Hydraulic Pressure Sensor/LConn1 -- A/RConn1
  Hydraulic Reference/LConn1 -- Hydraulic Pressure Sensor/RConn1

== system Brakes_Axle2_HydraulicValves_Channel4/HydraulicValves Channel4/Valves/Sensing pL1 ==
  Hydraulic Pressure Sensor : fl_lib/Isothermal Liquid/Sensors/Pressure Sensor (IL)  pressure_measure=foundation.enum.pressure_measure.difference
      settings: LibrarySourceBlock=|
      | fl_lib/Hydraulic/Hydraulic Sensors/Hydraulic Pressure
      | Sensor
  Hydraulic Reference : fl_lib/Isothermal Liquid/Elements/Reservoir (IL)  pressure_input=false  pressure_spec=foundation.enum.pressure_spec.atmospheric  reservoir_pressure=0.101325 MPa
      settings: LibrarySourceBlock=fl_lib/Hydraulic/Hydraulic Elements/Hydraulic Reference
  PS-Simulink Converter : nesl_utility/PS-Simulink Converter  PhysicalDomain=network_engine_domain  SubClassName=ps_output  LeftPortType=input  RightPortType=output  PseudoPeriodic=off  Frequencies=[]  VectorFormat=1-D array  Unit=bar  AffineConversion=off
  A : PMIOPort  Side=Left
  p : Outport  VectorParamsAs1DForOutWhenUnconnected=off
  wires:
  PS-Simulink Converter/1 -> p/1
  connections:
  Hydraulic Reference/LConn1 -- Hydraulic Pressure Sensor/RConn1
  Hydraulic Pressure Sensor/LConn1 -- A/RConn1
  Hydraulic Pressure Sensor/RConn2 -- PS-Simulink Converter/LConn1

== system Brakes_Axle2_HydraulicValves_Channel4/HydraulicValves Channel4/Valves/Sensing pRL ==
  Hydraulic Pressure Sensor : fl_lib/Isothermal Liquid/Sensors/Pressure Sensor (IL)  pressure_measure=foundation.enum.pressure_measure.difference
      settings: LibrarySourceBlock=|
      | fl_lib/Hydraulic/Hydraulic Sensors/Hydraulic Pressure
      | Sensor
  Hydraulic Reference : fl_lib/Isothermal Liquid/Elements/Reservoir (IL)  pressure_input=false  pressure_spec=foundation.enum.pressure_spec.atmospheric  reservoir_pressure=0.101325 MPa
      settings: LibrarySourceBlock=fl_lib/Hydraulic/Hydraulic Elements/Hydraulic Reference
  PS-Simulink Converter : nesl_utility/PS-Simulink Converter  PhysicalDomain=network_engine_domain  SubClassName=ps_output  LeftPortType=input  RightPortType=output  PseudoPeriodic=off  Frequencies=[]  VectorFormat=1-D array  Unit=bar  AffineConversion=off
  A : PMIOPort  Side=Left
  p : Outport  VectorParamsAs1DForOutWhenUnconnected=off
  wires:
  PS-Simulink Converter/1 -> p/1
  connections:
  Hydraulic Pressure Sensor/RConn2 -- PS-Simulink Converter/LConn1
  Hydraulic Pressure Sensor/LConn1 -- A/RConn1
  Hydraulic Reference/LConn1 -- Hydraulic Pressure Sensor/RConn1

== system Brakes_Axle2_HydraulicValves_Channel4/HydraulicValves Channel4/Valves/Sensing pRR ==
  Hydraulic Pressure Sensor : fl_lib/Isothermal Liquid/Sensors/Pressure Sensor (IL)  pressure_measure=foundation.enum.pressure_measure.difference
      settings: LibrarySourceBlock=|
      | fl_lib/Hydraulic/Hydraulic Sensors/Hydraulic Pressure
      | Sensor
  Hydraulic Reference : fl_lib/Isothermal Liquid/Elements/Reservoir (IL)  pressure_input=false  pressure_spec=foundation.enum.pressure_spec.atmospheric  reservoir_pressure=0.101325 MPa
      settings: LibrarySourceBlock=fl_lib/Hydraulic/Hydraulic Elements/Hydraulic Reference
  PS-Simulink Converter : nesl_utility/PS-Simulink Converter  PhysicalDomain=network_engine_domain  SubClassName=ps_output  LeftPortType=input  RightPortType=output  PseudoPeriodic=off  Frequencies=[]  VectorFormat=1-D array  Unit=bar  AffineConversion=off
  A : PMIOPort  Side=Left
  p : Outport  VectorParamsAs1DForOutWhenUnconnected=off
  wires:
  PS-Simulink Converter/1 -> p/1
  connections:
  Hydraulic Reference/LConn1 -- Hydraulic Pressure Sensor/RConn1
  Hydraulic Pressure Sensor/LConn1 -- A/RConn1
  Hydraulic Pressure Sensor/RConn2 -- PS-Simulink Converter/LConn1

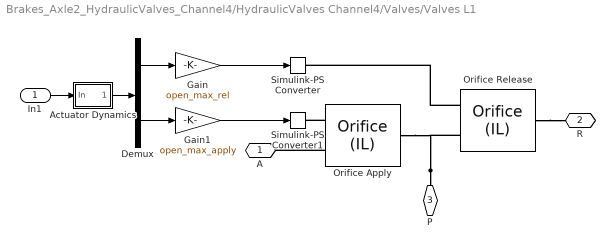
== system Brakes_Axle2_HydraulicValves_Channel4/HydraulicValves Channel4/Valves/Valves L1 ==
  In1 : Inport
  Actuator Dynamics : Subsystem  mask(First-order lag supporting vector signals){b=brkTs, x_initial=0}
      mask prompts: b "Filter time constant"; x_initial "Initial output"
      mask help: Models a lag of the form 1/(b*s+1) where s is the Laplace operator.
  Demux : Demux  Outputs=2
  Gain : Gain  Gain=open_max_rel
      settings: AttributesFormatString=%<Gain>
  Gain1 : Gain  Gain=open_max_apply
      settings: AttributesFormatString=%<Gain>
  Orifice Apply : SimscapeFluids_lib/Isothermal Liquid/Valves & Orifices/Orifices/Orifice (IL)  orifice_type=foundation.enum.constant_variable.variable  constant_orifice_spec=fluids.isothermal_liquid.valves_orifices.orifices.enum.constant_orifice_spec.area  variable_orifice_spec=1  orifice_area_constant=1e-3 m^2  p_diff_TLU_constant=[-4, -3, -2, -1, -.5, 0, .5, 1, 2, 3, 4] MPa  vol_flow_TLU_constant=[-2.44, -2.12, -1.68, -1.22, -.84, 0, .85, 1.21, 1.7, 2.09, 2.41] .* 1e-3 m^3/s  S_min=(open_max_apply)/(area_max_apply)*(1e-12) - (0) m  del_S=(-(0) + (open_max_apply)) - ((open_max_apply)/(area_max_apply)*(1e-12) - (0)) m  open_orientation=1  area_max=area_max_apply m^2  area_leak=1e-12 m^2  S_TLU=[-.002, 0, .002, .005, .015] - (0) m  orifice_area_TLU=[1e-09, 2.0352e-07, 4.0736e-05, .00011438, .00034356] m^2  area=inf m^2  Cd=0.7  Re_c=150  smoothing_factor=0  pressure_recovery=simscape.enum.onoff.off  S_vol_flow_TLU=[-.002, 0, .002, .005, .015] - (0) m  p_diff_TLU=[-10000000, -5000000, -2000000, 2000000, 5000000, 10000000] Pa  vol_flow_TLU=[-1e-07, -7.0711e-08, -4.4721e-08, 4.4721e-08, 7.0711e-08, 1e-07; -2.0352e-05, -1.4391e-05, -9.1017e-06, 9.1017e-06, 1.4391e-05, 2.0352e-05; -.0040736, -.0028805, -.0018218, .0018218, .0028805, .0040736; -.011438, -.0080879, -.0051152, .0051152, .0080879, .011438; -.034356, -.024293, -.015364, .015364, .024293, .034356] m^3/s
      settings: LibrarySourceBlock=sh_lib/Orifices/Variable Orifice
  Orifice Release : SimscapeFluids_lib/Isothermal Liquid/Valves & Orifices/Orifices/Orifice (IL)  orifice_type=foundation.enum.constant_variable.variable  constant_orifice_spec=fluids.isothermal_liquid.valves_orifices.orifices.enum.constant_orifice_spec.area  variable_orifice_spec=1  orifice_area_constant=1e-3 m^2  p_diff_TLU_constant=[-4, -3, -2, -1, -.5, 0, .5, 1, 2, 3, 4] MPa  vol_flow_TLU_constant=[-2.44, -2.12, -1.68, -1.22, -.84, 0, .85, 1.21, 1.7, 2.09, 2.41] .* 1e-3 m^3/s  S_min=(open_max_rel)/(area_max_rel)*(1e-12) - (0) m  del_S=(-(0) + (open_max_rel)) - ((open_max_rel)/(area_max_rel)*(1e-12) - (0)) m  open_orientation=1  area_max=area_max_rel m^2  area_leak=1e-12 m^2  S_TLU=[-.002, 0, .002, .005, .015] - (0) m  orifice_area_TLU=[1e-09, 2.0352e-07, 4.0736e-05, .00011438, .00034356] m^2  area=inf m^2  Cd=0.7  Re_c=150  smoothing_factor=0  pressure_recovery=simscape.enum.onoff.off  S_vol_flow_TLU=[-.002, 0, .002, .005, .015] - (0) m  p_diff_TLU=[-10000000, -5000000, -2000000, 2000000, 5000000, 10000000] Pa  vol_flow_TLU=[-1e-07, -7.0711e-08, -4.4721e-08, 4.4721e-08, 7.0711e-08, 1e-07; -2.0352e-05, -1.4391e-05, -9.1017e-06, 9.1017e-06, 1.4391e-05, 2.0352e-05; -.0040736, -.0028805, -.0018218, .0018218, .0028805, .0040736; -.011438, -.0080879, -.0051152, .0051152, .0080879, .011438; -.034356, -.024293, -.015364, .015364, .024293, .034356] m^3/s
      settings: LibrarySourceBlock=sh_lib/Orifices/Variable Orifice
  Simulink-PS Converter : nesl_utility/Simulink-PS Converter  PhysicalDomain=network_engine_domain  SubClassName=ps_input  LeftPortType=input  RightPortType=output  PseudoPeriodic=off  Frequencies=[]  NoiseDistribution=none  NoiseParameters=[]  Unit=1  AffineConversion=off  FilteringAndDerivatives=provide  SimscapeFilterOrder=1  InputFilterTimeConstant=0.001  UdotUserProvided=0
  Simulink-PS Converter1 : nesl_utility/Simulink-PS Converter  PhysicalDomain=network_engine_domain  SubClassName=ps_input  LeftPortType=input  RightPortType=output  PseudoPeriodic=off  Frequencies=[]  NoiseDistribution=none  NoiseParameters=[]  Unit=1  AffineConversion=off  FilteringAndDerivatives=provide  SimscapeFilterOrder=1  InputFilterTimeConstant=0.001  UdotUserProvided=0
  A : PMIOPort  Side=Left
  R : PMIOPort  Port=2  Side=Left
  P : PMIOPort  Port=3  Side=Right
  wires:
  Actuator Dynamics/1(Out) -> Demux/1
  Demux/2 -> Gain1/1
  Demux/1 -> Gain/1
  In1/1 -> Actuator Dynamics/1(In)
  Gain/1 -> Simulink-PS Converter/1
  Gain1/1 -> Simulink-PS Converter1/1
  connections:
  P/RConn1 -- Orifice Release/LConn1 -- Orifice Apply/RConn1
  Orifice Apply/LConn2 -- Simulink-PS Converter1/RConn1
  Orifice Apply/LConn1 -- A/RConn1
  Orifice Release/LConn2 -- Simulink-PS Converter/RConn1
  Orifice Release/RConn1 -- R/RConn1

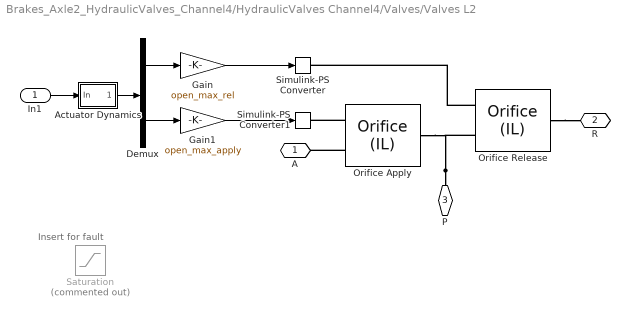
== system Brakes_Axle2_HydraulicValves_Channel4/HydraulicValves Channel4/Valves/Valves L2 ==
  note: Insert for fault
  In1 : Inport
  Actuator Dynamics : Subsystem  mask(First-order lag supporting vector signals){b=brkTs, x_initial=0}
      mask prompts: b "Filter time constant"; x_initial "Initial output"
      mask help: Models a lag of the form 1/(b*s+1) where s is the Laplace operator.
  Demux : Demux  Outputs=2
  Gain : Gain  Gain=open_max_rel
      settings: AttributesFormatString=%<Gain>
  Gain1 : Gain  Gain=open_max_apply
      settings: AttributesFormatString=%<Gain>
  Orifice Apply : SimscapeFluids_lib/Isothermal Liquid/Valves & Orifices/Orifices/Orifice (IL)  orifice_type=foundation.enum.constant_variable.variable  constant_orifice_spec=fluids.isothermal_liquid.valves_orifices.orifices.enum.constant_orifice_spec.area  variable_orifice_spec=1  orifice_area_constant=1e-3 m^2  p_diff_TLU_constant=[-4, -3, -2, -1, -.5, 0, .5, 1, 2, 3, 4] MPa  vol_flow_TLU_constant=[-2.44, -2.12, -1.68, -1.22, -.84, 0, .85, 1.21, 1.7, 2.09, 2.41] .* 1e-3 m^3/s  S_min=(open_max_apply)/(area_max_apply)*(1e-12) - (0) m  del_S=(-(0) + (open_max_apply)) - ((open_max_apply)/(area_max_apply)*(1e-12) - (0)) m  open_orientation=1  area_max=area_max_apply m^2  area_leak=1e-12 m^2  S_TLU=[-.002, 0, .002, .005, .015] - (0) m  orifice_area_TLU=[1e-09, 2.0352e-07, 4.0736e-05, .00011438, .00034356] m^2  area=inf m^2  Cd=0.7  Re_c=150  smoothing_factor=0  pressure_recovery=simscape.enum.onoff.off  S_vol_flow_TLU=[-.002, 0, .002, .005, .015] - (0) m  p_diff_TLU=[-10000000, -5000000, -2000000, 2000000, 5000000, 10000000] Pa  vol_flow_TLU=[-1e-07, -7.0711e-08, -4.4721e-08, 4.4721e-08, 7.0711e-08, 1e-07; -2.0352e-05, -1.4391e-05, -9.1017e-06, 9.1017e-06, 1.4391e-05, 2.0352e-05; -.0040736, -.0028805, -.0018218, .0018218, .0028805, .0040736; -.011438, -.0080879, -.0051152, .0051152, .0080879, .011438; -.034356, -.024293, -.015364, .015364, .024293, .034356] m^3/s
      settings: LibrarySourceBlock=sh_lib/Orifices/Variable Orifice
  Orifice Release : SimscapeFluids_lib/Isothermal Liquid/Valves & Orifices/Orifices/Orifice (IL)  orifice_type=foundation.enum.constant_variable.variable  constant_orifice_spec=fluids.isothermal_liquid.valves_orifices.orifices.enum.constant_orifice_spec.area  variable_orifice_spec=1  orifice_area_constant=1e-3 m^2  p_diff_TLU_constant=[-4, -3, -2, -1, -.5, 0, .5, 1, 2, 3, 4] MPa  vol_flow_TLU_constant=[-2.44, -2.12, -1.68, -1.22, -.84, 0, .85, 1.21, 1.7, 2.09, 2.41] .* 1e-3 m^3/s  S_min=(open_max_rel)/(area_max_rel)*(1e-12) - (0) m  del_S=(-(0) + (open_max_rel)) - ((open_max_rel)/(area_max_rel)*(1e-12) - (0)) m  open_orientation=1  area_max=area_max_rel m^2  area_leak=1e-12 m^2  S_TLU=[-.002, 0, .002, .005, .015] - (0) m  orifice_area_TLU=[1e-09, 2.0352e-07, 4.0736e-05, .00011438, .00034356] m^2  area=inf m^2  Cd=0.7  Re_c=150  smoothing_factor=0  pressure_recovery=simscape.enum.onoff.off  S_vol_flow_TLU=[-.002, 0, .002, .005, .015] - (0) m  p_diff_TLU=[-10000000, -5000000, -2000000, 2000000, 5000000, 10000000] Pa  vol_flow_TLU=[-1e-07, -7.0711e-08, -4.4721e-08, 4.4721e-08, 7.0711e-08, 1e-07; -2.0352e-05, -1.4391e-05, -9.1017e-06, 9.1017e-06, 1.4391e-05, 2.0352e-05; -.0040736, -.0028805, -.0018218, .0018218, .0028805, .0040736; -.011438, -.0080879, -.0051152, .0051152, .0080879, .011438; -.034356, -.024293, -.015364, .015364, .024293, .034356] m^3/s
      settings: LibrarySourceBlock=sh_lib/Orifices/Variable Orifice
  Saturation : Saturate  Commented=on  UpperLimit=inf  LowerLimit=0.5
  Simulink-PS Converter : nesl_utility/Simulink-PS Converter  PhysicalDomain=network_engine_domain  SubClassName=ps_input  LeftPortType=input  RightPortType=output  PseudoPeriodic=off  Frequencies=[]  NoiseDistribution=none  NoiseParameters=[]  Unit=1  AffineConversion=off  FilteringAndDerivatives=provide  SimscapeFilterOrder=1  InputFilterTimeConstant=0.001  UdotUserProvided=0
  Simulink-PS Converter1 : nesl_utility/Simulink-PS Converter  PhysicalDomain=network_engine_domain  SubClassName=ps_input  LeftPortType=input  RightPortType=output  PseudoPeriodic=off  Frequencies=[]  NoiseDistribution=none  NoiseParameters=[]  Unit=1  AffineConversion=off  FilteringAndDerivatives=provide  SimscapeFilterOrder=1  InputFilterTimeConstant=0.001  UdotUserProvided=0
  A : PMIOPort  Side=Left
  R : PMIOPort  Port=2  Side=Left
  P : PMIOPort  Port=3  Side=Right
  wires:
  In1/1 -> Actuator Dynamics/1(In)
  Actuator Dynamics/1(Out) -> Demux/1
  Demux/1 -> Gain/1
  Gain/1 -> Simulink-PS Converter/1
  Gain1/1 -> Simulink-PS Converter1/1
  Demux/2 -> Gain1/1
  connections:
  Orifice Apply/LConn2 -- Simulink-PS Converter1/RConn1
  Orifice Apply/LConn1 -- A/RConn1
  P/RConn1 -- Orifice Release/LConn1 -- Orifice Apply/RConn1
  Orifice Release/LConn2 -- Simulink-PS Converter/RConn1
  Orifice Release/RConn1 -- R/RConn1

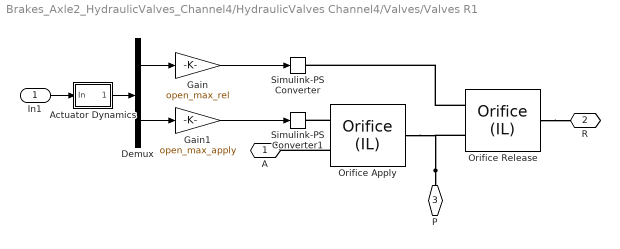
== system Brakes_Axle2_HydraulicValves_Channel4/HydraulicValves Channel4/Valves/Valves R1 ==
  In1 : Inport
  Actuator Dynamics : Subsystem  mask(First-order lag supporting vector signals){b=brkTs, x_initial=0}
      mask prompts: b "Filter time constant"; x_initial "Initial output"
      mask help: Models a lag of the form 1/(b*s+1) where s is the Laplace operator.
  Demux : Demux  Outputs=2
  Gain : Gain  Gain=open_max_rel
      settings: AttributesFormatString=%<Gain>
  Gain1 : Gain  Gain=open_max_apply
      settings: AttributesFormatString=%<Gain>
  Orifice Apply : SimscapeFluids_lib/Isothermal Liquid/Valves & Orifices/Orifices/Orifice (IL)  orifice_type=foundation.enum.constant_variable.variable  constant_orifice_spec=fluids.isothermal_liquid.valves_orifices.orifices.enum.constant_orifice_spec.area  variable_orifice_spec=1  orifice_area_constant=1e-3 m^2  p_diff_TLU_constant=[-4, -3, -2, -1, -.5, 0, .5, 1, 2, 3, 4] MPa  vol_flow_TLU_constant=[-2.44, -2.12, -1.68, -1.22, -.84, 0, .85, 1.21, 1.7, 2.09, 2.41] .* 1e-3 m^3/s  S_min=(open_max_apply)/(area_max_apply)*(1e-12) - (0) m  del_S=(-(0) + (open_max_apply)) - ((open_max_apply)/(area_max_apply)*(1e-12) - (0)) m  open_orientation=1  area_max=area_max_apply m^2  area_leak=1e-12 m^2  S_TLU=[-.002, 0, .002, .005, .015] - (0) m  orifice_area_TLU=[1e-09, 2.0352e-07, 4.0736e-05, .00011438, .00034356] m^2  area=inf m^2  Cd=0.7  Re_c=150  smoothing_factor=0  pressure_recovery=simscape.enum.onoff.off  S_vol_flow_TLU=[-.002, 0, .002, .005, .015] - (0) m  p_diff_TLU=[-10000000, -5000000, -2000000, 2000000, 5000000, 10000000] Pa  vol_flow_TLU=[-1e-07, -7.0711e-08, -4.4721e-08, 4.4721e-08, 7.0711e-08, 1e-07; -2.0352e-05, -1.4391e-05, -9.1017e-06, 9.1017e-06, 1.4391e-05, 2.0352e-05; -.0040736, -.0028805, -.0018218, .0018218, .0028805, .0040736; -.011438, -.0080879, -.0051152, .0051152, .0080879, .011438; -.034356, -.024293, -.015364, .015364, .024293, .034356] m^3/s
      settings: LibrarySourceBlock=sh_lib/Orifices/Variable Orifice
  Orifice Release : SimscapeFluids_lib/Isothermal Liquid/Valves & Orifices/Orifices/Orifice (IL)  orifice_type=foundation.enum.constant_variable.variable  constant_orifice_spec=fluids.isothermal_liquid.valves_orifices.orifices.enum.constant_orifice_spec.area  variable_orifice_spec=1  orifice_area_constant=1e-3 m^2  p_diff_TLU_constant=[-4, -3, -2, -1, -.5, 0, .5, 1, 2, 3, 4] MPa  vol_flow_TLU_constant=[-2.44, -2.12, -1.68, -1.22, -.84, 0, .85, 1.21, 1.7, 2.09, 2.41] .* 1e-3 m^3/s  S_min=(open_max_rel)/(area_max_rel)*(1e-12) - (0) m  del_S=(-(0) + (open_max_rel)) - ((open_max_rel)/(area_max_rel)*(1e-12) - (0)) m  open_orientation=1  area_max=area_max_rel m^2  area_leak=1e-12 m^2  S_TLU=[-.002, 0, .002, .005, .015] - (0) m  orifice_area_TLU=[1e-09, 2.0352e-07, 4.0736e-05, .00011438, .00034356] m^2  area=inf m^2  Cd=0.7  Re_c=150  smoothing_factor=0  pressure_recovery=simscape.enum.onoff.off  S_vol_flow_TLU=[-.002, 0, .002, .005, .015] - (0) m  p_diff_TLU=[-10000000, -5000000, -2000000, 2000000, 5000000, 10000000] Pa  vol_flow_TLU=[-1e-07, -7.0711e-08, -4.4721e-08, 4.4721e-08, 7.0711e-08, 1e-07; -2.0352e-05, -1.4391e-05, -9.1017e-06, 9.1017e-06, 1.4391e-05, 2.0352e-05; -.0040736, -.0028805, -.0018218, .0018218, .0028805, .0040736; -.011438, -.0080879, -.0051152, .0051152, .0080879, .011438; -.034356, -.024293, -.015364, .015364, .024293, .034356] m^3/s
      settings: LibrarySourceBlock=sh_lib/Orifices/Variable Orifice
  Simulink-PS Converter : nesl_utility/Simulink-PS Converter  PhysicalDomain=network_engine_domain  SubClassName=ps_input  LeftPortType=input  RightPortType=output  PseudoPeriodic=off  Frequencies=[]  NoiseDistribution=none  NoiseParameters=[]  Unit=1  AffineConversion=off  FilteringAndDerivatives=provide  SimscapeFilterOrder=1  InputFilterTimeConstant=0.001  UdotUserProvided=0
  Simulink-PS Converter1 : nesl_utility/Simulink-PS Converter  PhysicalDomain=network_engine_domain  SubClassName=ps_input  LeftPortType=input  RightPortType=output  PseudoPeriodic=off  Frequencies=[]  NoiseDistribution=none  NoiseParameters=[]  Unit=1  AffineConversion=off  FilteringAndDerivatives=provide  SimscapeFilterOrder=1  InputFilterTimeConstant=0.001  UdotUserProvided=0
  A : PMIOPort  Side=Left
  R : PMIOPort  Port=2  Side=Left
  P : PMIOPort  Port=3  Side=Right
  wires:
  Actuator Dynamics/1(Out) -> Demux/1
  In1/1 -> Actuator Dynamics/1(In)
  Demux/1 -> Gain/1
  Gain/1 -> Simulink-PS Converter/1
  Gain1/1 -> Simulink-PS Converter1/1
  Demux/2 -> Gain1/1
  connections:
  Orifice Apply/LConn2 -- Simulink-PS Converter1/RConn1
  Orifice Apply/LConn1 -- A/RConn1
  P/RConn1 -- Orifice Release/LConn1 -- Orifice Apply/RConn1
  Orifice Release/LConn2 -- Simulink-PS Converter/RConn1
  Orifice Release/RConn1 -- R/RConn1
